simulink model "formation_control"  (R2021a)
settings: Solver=VariableStepAuto  StartTime=0.0  StopTime=T  RelTol=1e-3
undefined symbols (not defined in the file or in its folder): params
settings Model: Creator=gaeta  LastModifiedBy=giuse
settings SolverCC: AlgebraicLoopSolver=TrustRegion
settings DataIOCC: InitialState=initialCondition  LoadInitialState=on
settings DebuggingCC: SFMachineParentedDataDiag=warning

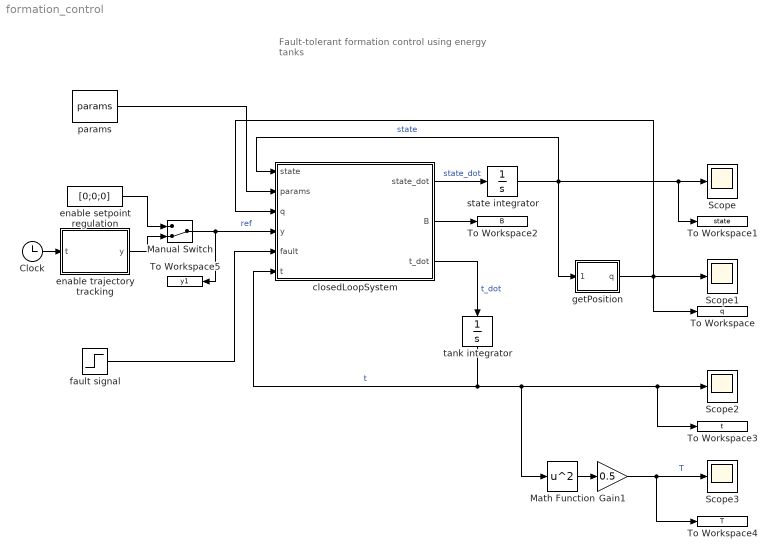
== system formation_control ==
  note: Fault-tolerant formation control
      | using energy tanks
  Clock : Clock
  Gain1 : Gain  Gain=0.5
  Manual Switch : ManualSwitch  CurrentSetting=0
  Math Function : Math  Operator=square  SaturateOnIntegerOverflow=on
  Scope{,1..3} (4 alike) : Scope
  To Workspace : ToWorkspace  VariableName=q  SaveFormat=Timeseries  SampleTime=-1
  To Workspace1 : ToWorkspace  VariableName=state  SaveFormat=Timeseries  SampleTime=-1
  To Workspace2 : ToWorkspace  VariableName=B  SaveFormat=Timeseries  SampleTime=-1
  To Workspace3 : ToWorkspace  VariableName=t  SaveFormat=Timeseries  SampleTime=-1
  To Workspace4 : ToWorkspace  VariableName=T  SaveFormat=Timeseries  SampleTime=-1
  To Workspace5 : ToWorkspace  VariableName=y1  SaveFormat=Timeseries  SampleTime=-1
  closedLoopSystem : MATLAB Function  TreatAsAtomicUnit=on
  enable setpoint regulation : Constant  Value=[0;0;0]
  enable trajectory tracking : MATLAB Function  TreatAsAtomicUnit=on
  fault signal : Step  Time=40  SampleTime=0
  getPosition : Subsystem
  params : Constant  Value=params  OutDataTypeStr=Bus: params_bus
  state integrator : Integrator
  tank integrator : Integrator
  wires:
  params/1 -> closedLoopSystem/2(params)
  state integrator/1 -> To Workspace1/1, Scope/1, closedLoopSystem/1(state), getPosition/1(state)  "state"
  closedLoopSystem/1(state_dot) -> state integrator/1  "state_dot"
  getPosition/1(q) -> To Workspace/1, Scope1/1, closedLoopSystem/3(q)
  closedLoopSystem/2(B) -> To Workspace2/1
  closedLoopSystem/3(t_dot) -> tank integrator/1  "t_dot"
  tank integrator/1 -> Math Function/1, To Workspace3/1, Scope2/1, closedLoopSystem/6(t)  "t"
  Math Function/1 -> Gain1/1
  Gain1/1 -> To Workspace4/1, Scope3/1  "T"
  enable trajectory tracking/1(y) -> Manual Switch/2
  fault signal/1 -> closedLoopSystem/5(fault)
  enable setpoint regulation/1 -> Manual Switch/1
  Clock/1 -> enable trajectory tracking/1(t)
  Manual Switch/1 -> closedLoopSystem/4(y), To Workspace5/1  "ref"

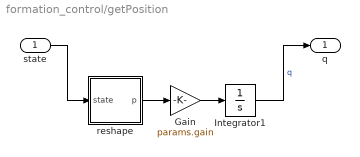
== system formation_control/getPosition ==
  state : Inport
  Gain : Gain  Gain=params.gain
  Integrator1 : Integrator
  reshape : MATLAB Function  TreatAsAtomicUnit=on
  q : Outport
  wires:
  state/1 -> reshape/1(state)
  reshape/1(p) -> Gain/1
  Gain/1 -> Integrator1/1
  Integrator1/1 -> q/1  "q"

== matlab function formation_control/enable trajectory tracking ==
  data: y output size=3; t input size=1
%% generate reference trajectory
function y = trajectory(t)
    t1 = 5;
    t_end = 100;
    
    w = 0.1;
    A = 80;
    z_vel = 0.8;
    
	if(t<t1)
        y = [0;0;0];
    elseif(t>t_end)
        y = [A*sin(w*t_end); -A*cos(w*t_end); z_vel*t_end] - [A*sin(w*t1); -A*cos(w*t1); z_vel*t1];
    else
        y = [A*sin(w*t); -A*cos(w*t); z_vel*t] - [A*sin(w*t1); -A*cos(w*t1); z_vel*t1];
    end
end

== matlab function formation_control/closedLoopSystem ==
  data: state input size=3*(params.N+params.E); state_dot output size=3*(params.N+params.E); params input; q input size=3*params.N; y input size=3; fault input; t input size=params.N; B output; t_dot output size=params.N
function [state_dot,B,t_dot] = closedLoopSystem(state, params, q, y, fault, t)
    n = 3;                      % task space
    N = params.N;               % number of robots
    
    %% initialize some matrices
    p = state(1:n*N);           % robots momenta
    m = params.m;               % robots masses
    M = zeros(n*N, n*N);      	% inertia matrix
    d = params.d;               % frict. coeff
    D = zeros(n*N, n*N);        % system dissipation matrix
    for i = 1:N
        M(n*i-n+1:n*i, n*i-n+1:n*i) = eye(n).*m(i);
        D(n*i-n+1:n*i, n*i-n+1:n*i) = eye(n).*d(i);
    end
    
    E = params.E;               % number of edges
    
    %% Check whether a fault is occurred
    if(sum(fault)~=0 && ~params.fault_occurred)
        params.fault_occurred = 1;  % flag on
        faulted_robot = 3;
        [params.B, params.joined_edge] = faultHandler(params.B, params.Bfull, faulted_robot);
    end
    
    %% Still initialize matrices
    B = params.B;
    Bcl = kron(params.B,eye(n));	% closed-loop incidence matrix    

    z = state(n*N+1:n*(N+E));	% edges lengths
    z_des = params.z_des;       % desired edges lengths
    dc = params.dc;             % robots dissipations
    Dc = zeros(n*E, n*E);       % controller dissipation matrix
    kc = params.kc;             % constant springs
    Kc = zeros(n*E, n*E);       % constant spring matrix
    for j = 1:E
        Dc(n*j-n+1:n*j, n*j-n+1:n*j) = eye(n).*dc(j);
        Kc(n*j-n+1:n*j, n*j-n+1:n*j) = eye(n).*kc(j);
    end
    
    % NOTE: constant matrices M, D, Dc, Kc should be moved in the Init file
    
    %% Energy transfer protocol
    
    t_dot = zeros(size(t));     % tanks dynamics
    w = zeros(E*n,1);           % additional input for energy transfer
    
    if(params.fault_occurred)  
        e = params.joined_edge;
        
        Fa_ij = zeros(n,1);
        for i = 1:n
           Fa_ij(i) = Vdot( z(e*n-n+i)-z_des(e*n-n+i) );
        end
           
        i = find(B(:,e)==-1);
        j = find(B(:,e)==1);
        
        Diss = p.'*(inv(M).'*D*inv(M))*p;       % energy dissipation
        
        %update tank i
        wt_ij = -params.gamma(e)*(Fa_ij.'*Fa_ij)*t(i);
        t_dot_i = Diss/t(i) + wt_ij;
        if( all(t(i)>params.tank_max & t_dot_i>0) || all(t(i)<params.tank_min & t_dot_i<0) )
            t_dot(i) = 0;
        else
            t_dot(i) = t_dot_i;
        end
        
        %update tank j
        wt_ji = -params.gamma(e)*(Fa_ij.'*Fa_ij)*t(j);
        t_dot_j = Diss/t(j) + wt_ji;
        if( all(t(j)>params.tank_max & t_dot_j>0) || all(t(j)<params.tank_min & t_dot_j<0) )
            t_dot(j) = 0;
        else
            t_dot(j) = t_dot_j;
        end
                    
        % update w
        wz_ij = -params.gamma(e)*Fa_ij*t(i)^2 - params.gamma(e)*Fa_ij*t(j)^2;
        w(e*n-n+1:e*n) = wz_ij;
    end
    
    %% Trajectory Tracking / Eetpoint Regulation
    tracking = true;    % #CHANGE THIS: ENABLE/DISABLE TRAJECTORY TRACKING
    u = zeros(n,1);
    if(tracking)
        Kp = 25;
        u = Kp*(y-q(1:n)); % control for trajectory tracking 
    end
    
    %% Multi-robot System Dynamics
    Fe = -Bcl * Kc*(z-z_des);           % external forces (control action)
    Fa = -(Bcl*Dc*Bcl.')*(M^(-1)*p);    % interaction (coupling) forces
    p_dot = Fa + Fe - D*(M^(-1)*p) + [u; zeros(n*(N-1),1)];
    z_dot = Bcl.'*(M^(-1)*p) + w;
    state_dot = [p_dot; z_dot];
   
end


%% Potential energy function
function v = V(error)
	if (error<=0)
        v = error^2;
    elseif(error>=0 && error<5*pi)
        v = 50*cos(0.2*error-pi)+50;
    else
        v = 100;
    end
end

%% Derivative of the Potential energy function
function vdot = Vdot(error)
    if (error<=0)
        vdot = 2*error;
    elseif(error>0 && error<5*pi)
        vdot = 10*sin(0.2*error);
    else
        vdot = 0;
    end
end

%% Split & Join operations
function [B, joined_edge] = faultHandler(B, Bfull, faulted_robot)
    % split 
    if(faulted_robot==1)
        disp("leader cannot be faulted by hypothesis");
    else
        z = zeros(size(B,1),2);
        B = [B(:, 1:faulted_robot-2), z, B(:, faulted_robot+1:size(B,2))];
        B(faulted_robot,:) = zeros(1, size(B,2));
    end
    
    % join
    N = size(B,1);
    if(faulted_robot==N)
        r1 = faulted_robot-1;
        r2 = 1;
    else
        r1 = faulted_robot-1;
        r2 = faulted_robot+1;
    end
	for e = 1:size(Bfull,2)
        if( (Bfull(r1,e)==1 && Bfull(r2,e)==-1) || (Bfull(r1,e)==-1 && Bfull(r2,e)==1) )
            B(:,e) = Bfull(:,e);
            break
        end
    end
    joined_edge = e;
end


%

== matlab function formation_control/getPosition/reshape ==
  data: p output size=params.N*3; state input
function p = reshape(state)
    n = 3;
    %N = roots([n/2, n/2, -size(state,1)]).'*(roots([n/2, n/2, -size(state,1)])>0);
    N = 5;
    p = state(1:3*N);
end




%
